simulink model "lab4"  (R2022b)
settings: Solver=VariableStepAuto  StartTime=0.0  StopTime=10.0  RelTol=1e-3
values from neighbouring files (symbols this model uses):
  m1 = str2num(get_param("lab4/Subsystem", "m1"))    [lab4_f.m]
undefined symbols (not defined in the file or in its folder): g, M, m2, R, r
settings Model: Creator=bm50345  LastModifiedBy=bm50345

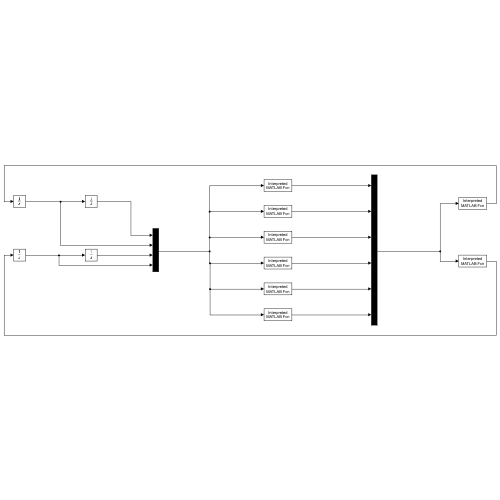
[thumbnail: Simulink's stored preview of the top-level diagram]
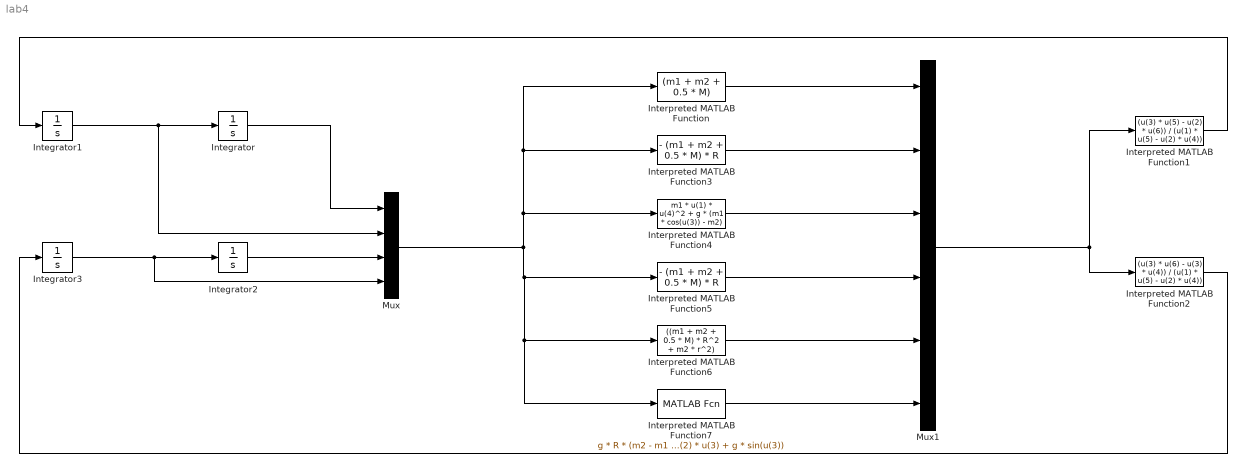
== system lab4 ==
  Integrator{,1..3} (4 alike) : Integrator
  Interpreted MATLAB Function : MATLABFcn  MATLABFcn=(m1 + m2 + 0.5 * M)
  Interpreted MATLAB Function1 : MATLABFcn  MATLABFcn=(u(3) * u(5) - u(2) * u(6)) / (u(1) * u(5) - u(2) * u(4))
  Interpreted MATLAB Function2 : MATLABFcn  MATLABFcn=(u(3) * u(6) - u(3) * u(4)) / (u(1) * u(5) - u(2) * u(4))
  Interpreted MATLAB Function3 : MATLABFcn  MATLABFcn=- (m1 + m2 + 0.5 * M) * R
  Interpreted MATLAB Function4 : MATLABFcn  MATLABFcn=m1 * u(1) * u(4)^2 + g * (m1 * cos(u(3)) - m2)
  Interpreted MATLAB Function5 : MATLABFcn  MATLABFcn=- (m1 + m2 + 0.5 * M) * R
  Interpreted MATLAB Function6 : MATLABFcn  MATLABFcn=((m1 + m2 + 0.5 * M) * R^2 + m2 * r^2)
  Interpreted MATLAB Function7 : MATLABFcn  MATLABFcn=g * R * (m2 - m1 * cos(u(3)) - m1 * r * (2 * u(2) * u(3) + g * sin(u(3))
  Mux : Mux
  Mux1 : Mux  Inputs=6
  wires:
  Mux1/1 -> Interpreted MATLAB Function1/1, Interpreted MATLAB Function2/1
  Integrator3/1 -> Mux/4, Integrator2/1
  Integrator1/1 -> Mux/2, Integrator/1
  Integrator2/1 -> Mux/3
  Integrator/1 -> Mux/1
  Interpreted MATLAB Function/1 -> Mux1/1
  Interpreted MATLAB Function3/1 -> Mux1/2
  Interpreted MATLAB Function4/1 -> Mux1/3
  Interpreted MATLAB Function5/1 -> Mux1/4
  Interpreted MATLAB Function6/1 -> Mux1/5
  Interpreted MATLAB Function7/1 -> Mux1/6
  Interpreted MATLAB Function2/1 -> Integrator3/1
  Interpreted MATLAB Function1/1 -> Integrator1/1
  Mux/1 -> Interpreted MATLAB Function/1, Interpreted MATLAB Function3/1, Interpreted MATLAB Function4/1, Interpreted MATLAB Function7/1, Interpreted MATLAB Function6/1, Interpreted MATLAB Function5/1
